simulink library "asbCubeSatSensorsLib"  (R2023b)
settings: Solver=VariableStepAuto  StartTime=0.0  StopTime=10.0  RelTol=1e-3
undefined symbols (not defined in the file): CubeSatTimeStep
libraries: simulink x1, sharedTrackingLibrary x1
settings Model: Creator=The MathWorks, Inc.  LastModifiedBy=bobow
settings SolverCC: AlgebraicLoopSolver=TrustRegion  MaxZcPerStep=1
settings DataIOCC: ReturnWorkspaceOutputs=off
settings DebuggingCC: UnconnectedInputMsg=warning  UnconnectedOutputMsg=warning  UnconnectedLineMsg=warning  ArithmeticOperatorsInVariantConditions=warning
settings ModelReferenceCC: EnableRefExpFcnMdlSchedulingChecks=on

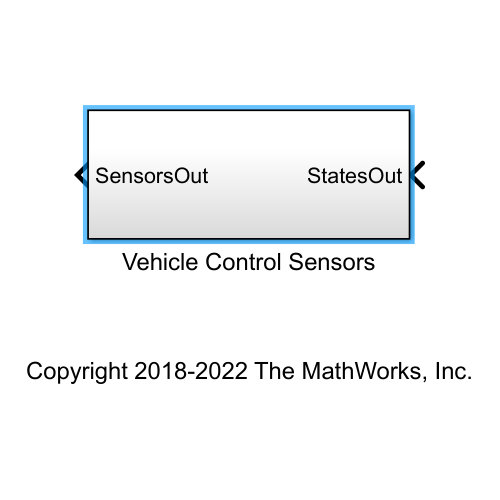
[thumbnail: Simulink's stored preview of the top-level diagram]
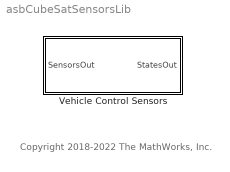
== system asbCubeSatSensorsLib ==
  note: Copyright 2018-2022 The MathWorks, Inc.
  Vehicle Control Sensors : Subsystem  RequirementInfo={} %GIDa_45822218_a1a7_4b71_b24f_41bd1b8f625c

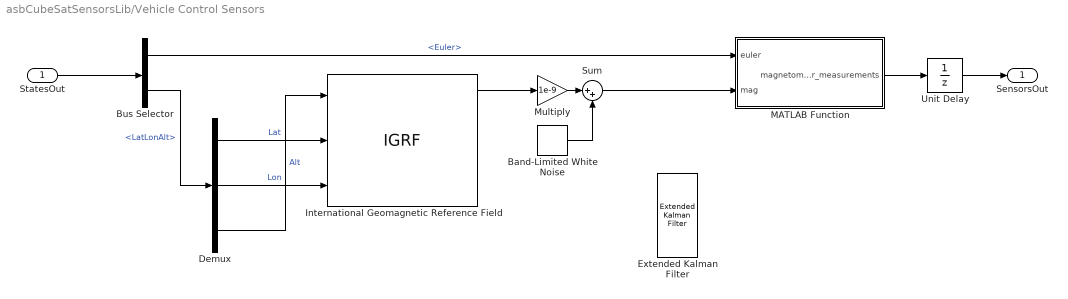
== system asbCubeSatSensorsLib/Vehicle Control Sensors ==
  StatesOut : Inport  RequirementInfo={} %GIDa_90530906_86a2_4375_ad60_16b58fab3a32  OutDataTypeStr=Bus: StatesOutBus
  Band-Limited White Noise : simulink/Sources/Band-Limited White Noise  Cov=3e-8*[1,1,1]  Ts=CubeSatTimeStep  seed=[23341]
  Bus Selector : BusSelector  OutputSignals=Euler,LatLonAlt
  Demux : Demux  Outputs=3
  Extended Kalman Filter : sharedTrackingLibrary/Extended Kalman Filter  StateTransitionFcn=myStateTransitionFcn  HasStateTransitionJacobianFcn=off  HasAdditiveProcessNoise=Additive  ProcessNoise=1  HasTimeVaryingProcessNoise=off  HasStateTransitionFcnExtraArgument=0  InitialState=0  InitialStateCovariance=1  MeasurementFcn1=myMeasurementFcn  HasMeasurementJacobianFcn1=off  HasMeasurementEnablePort1=off  HasAdditiveMeasurementNoise1=Additive  MeasurementNoise1=1  HasTimeVaryingMeasurementNoise1=off  HasMeasurementFcnExtraArgument1=0  HasMeasurementWrapping1=off  MeasurementFcn2=myMeasurementFcn  HasMeasurementJacobianFcn2=off  HasMeasurementEnablePort2=off  HasAdditiveMeasurementNoise2=Additive  MeasurementNoise2=1  HasTimeVaryingMeasurementNoise2=off  HasMeasurementFcnExtraArgument2=0  HasMeasurementWrapping2=off  MeasurementFcn3=myMeasurementFcn  HasMeasurementJacobianFcn3=off  HasMeasurementEnablePort3=off  HasAdditiveMeasurementNoise3=Additive  MeasurementNoise3=1  HasTimeVaryingMeasurementNoise3=off  HasMeasurementFcnExtraArgument3=0  HasMeasurementWrapping3=off  MeasurementFcn4=myMeasurementFcn  HasMeasurementJacobianFcn4=off  HasMeasurementEnablePort4=off  HasAdditiveMeasurementNoise4=Additive  MeasurementNoise4=1  HasTimeVaryingMeasurementNoise4=off  HasMeasurementFcnExtraArgument4=0  HasMeasurementWrapping4=off  MeasurementFcn5=myMeasurementFcn  HasMeasurementJacobianFcn5=off  HasMeasurementEnablePort5=off  HasAdditiveMeasurementNoise5=Additive  MeasurementNoise5=1  HasTimeVaryingMeasurementNoise5=off  HasMeasurementFcnExtraArgument5=0  HasMeasurementWrapping5=off  EnableMultirate=off  StateTransitionFcnSampleTime=1  MeasurementFcn1SampleTime=1  MeasurementFcn2SampleTime=1  MeasurementFcn3SampleTime=1  MeasurementFcn4SampleTime=1  MeasurementFcn5SampleTime=1  UseCurrentEstimator=on  OutputStateCovariance=off  DataType=double  SampleTime=1  NumberOfMeasurements=1
  International Geomagnetic Reference Field : IGRF  time_in=off  month=January  day=1  year=2020  sv_out=off
      settings: AttributesFormatString=%<generation>
  MATLAB Function : MATLAB Function  TreatAsAtomicUnit=on
  Multiply : Gain  Gain=1e-9
  Sum : Sum  Inputs=|++
  Unit Delay : UnitDelay  RequirementInfo={} %GIDa_09aaba6b_aadd_457c_a1ec_e9b9a273eb2e  SampleTime=CubeSatTimeStep  HasFrameUpgradeWarning=on
  SensorsOut : Outport  RequirementInfo={} %GIDa_3b6c2e72_aaee_4cf6_9430_15b046ac2608  OutDataTypeStr=double  VectorParamsAs1DForOutWhenUnconnected=off
  wires:
  Sum/1 -> MATLAB Function/2(mag)
  Band-Limited White Noise/1 -> Sum/2
  MATLAB Function/1(magnetometer_measurements) -> Unit Delay/1
  Multiply/1 -> Sum/1
  Bus Selector/1 -> MATLAB Function/1(euler)  "<Euler>"
  International Geomagnetic Reference Field/1 -> Multiply/1
  Demux/3 -> International Geomagnetic Reference Field/1  "Alt"
  Demux/2 -> International Geomagnetic Reference Field/3  "Lon"
  Demux/1 -> International Geomagnetic Reference Field/2  "Lat"
  Bus Selector/2 -> Demux/1  "<LatLonAlt>"
  StatesOut/1 -> Bus Selector/1
  Unit Delay/1 -> SensorsOut/1

== matlab function asbCubeSatSensorsLib/Vehicle Control Sensors/MATLAB Function ==
  data: euler input; magnetometer_measurements output; mag input
function magnetometer_measurements = fcn(euler, mag)
    q = quaternion(euler', 'eulerd', 'zyx', 'frame');
    magnetometer_measurements = rotateframe(q, mag');
